simulink library "avl2DLiftingBdy_cl"  (R2018b)
settings: Solver=VariableStepAuto  StartTime=0.0  StopTime=10.0  RelTol=1e-3
values from neighbouring files (symbols this model uses):
  Bref = dsgnData.Bref    [avl2DLiftingBdy_ts.m]
  Cref = dsgnData.Cref    [avl2DLiftingBdy_ts.m]
  grav = 9.81    [avl2DLiftingBdy_ts.m]
  ini_euler = [0;0;0]    [avl2DLiftingBdy_ts.m]
  ini_O_Vcm_o = [0;0;0]    [avl2DLiftingBdy_ts.m]
  ini_OwB = [0;0;0]    [avl2DLiftingBdy_ts.m]
  ini_Rcm_o = [0;0;0]    [avl2DLiftingBdy_ts.m]
  mass = 10    [avl2DLiftingBdy_ts.m]
  MI = eye(3)    [avl2DLiftingBdy_ts.m]
  Rcb_cm = [0;0;0.1]    [avl2DLiftingBdy_ts.m]
  rho_fluid = 1    [avl2DLiftingBdy_ts.m]
  Sref = dsgnData.Sref    [avl2DLiftingBdy_ts.m]
  vol = 20    [avl2DLiftingBdy_ts.m]
undefined symbols (not defined in the file or in its folder): CDtot_2D_Tbl, CLtot_2D_Tbl, Cltot_2D_Tbl, Cmtot_2D_Tbl, Cntot_2D_Tbl, k_CS_gain, m_added, some_class, turbine
libraries: BdyFrameGravForce_ul x1, avlAerodynamics2D x1, bdyFrameBuoyFnM_ul x1, calcAttchPtStates_ul x1, simpleDragTurbine_ul x1, sixDoFDynamics_ul x1, sumAttchPtsFnM_ul x1
settings Model: Creator=Ayaz  LastModifiedBy=asiddiq2

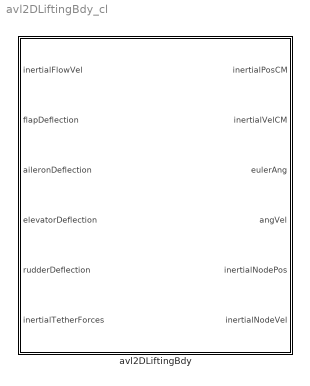
== system avl2DLiftingBdy_cl ==
  avl2DLiftingBdy : Subsystem  mask{M=mass, M_added=m_added, J=MI, vol=vol, Rcb_cm=Rcb_cm, turb_struct=turbine, cls_obj=some_class, g=grav, rho_fluid=rho_fluid, initPos=ini_Rcm_o, initVel=ini_O_Vcm_o, initEulAngs=ini_euler, initAngVel=ini_OwB, CLTable=CLtot_2D_Tbl, CDTable=CDtot_2D_Tbl, CMxTable=Cltot_2D_Tbl, CMyTable=Cmtot_2D_Tbl, CMzTable=Cntot_2D_Tbl, CsGainMatrix=k_CS_gain, CRef=Cref, BRef=Bref, SRef=Sref}
      mask prompts: M "Mass"; M_added "Added Mass Matrix"; J "Inertia matrix"; vol "Body volume"; Rcb_cm "Center of buoyamcy vector"; turb_struct "Turbines structure"; cls_obj "Object consisting variable '.tetherAttchPt'"; g "Gravitational acceleration"; rho_fluid "Fluid density"; initPos "Initial position"; initVel "Initial velocity"; initEulAngs "Initial Euler Angles"; initAngVel "Initial Angular Velocity Vec"; CLTable "CL lookup table object"; CDTable "CD lookup table object"; CMxTable "CMx lookup table object"; CMyTable "CMy lookup table object"; CMzTable "CMz lookup table object"; CsGainMatrix "Control surface gain matrix"; CRef "Pitch Moment Reference Length (AVL Cref)"; BRef "Roll & Yaw Moment Reference Length (AVL Bref)"; SRef "Ref area (AVL Sref)"
      mask TypeOptions M: BdyFrameGravForce/M | sixDoFDynamics1/M
      mask TypeOptions M_added: sixDoFDynamics1/M_added
      mask TypeOptions J: sixDoFDynamics1/J
      mask TypeOptions vol: bdyFrameBuoyForceAndMoment/vol
      mask TypeOptions Rcb_cm: bdyFrameBuoyForceAndMoment/Rcb_cm
      mask TypeOptions turb_struct: simpleDragTurbine/turb_struct
      mask TypeOptions cls_obj: calcAttchPtStates/cls_obj | sumAttchPtsFnM/cls_obj
      mask TypeOptions g: BdyFrameGravForce/g | bdyFrameBuoyForceAndMoment/g
      mask TypeOptions rho_fluid: avlAerodynamics2D/rho_fluid | bdyFrameBuoyForceAndMoment/rho_fluid | simpleDragTurbine/rho_fluid
      mask TypeOptions initPos: sixDoFDynamics1/initPos
      mask TypeOptions initVel: sixDoFDynamics1/initVel
      mask TypeOptions initEulAngs: sixDoFDynamics1/initEulAngs
      mask TypeOptions initAngVel: sixDoFDynamics1/initAngVel
      mask TypeOptions CLTable: avlAerodynamics2D/CLTable
      mask TypeOptions CDTable: avlAerodynamics2D/CDTable
      mask TypeOptions CMxTable: avlAerodynamics2D/CMxTable
      mask TypeOptions CMyTable: avlAerodynamics2D/CMyTable
      mask TypeOptions CMzTable: avlAerodynamics2D/CMzTable
      mask TypeOptions CsGainMatrix: avlAerodynamics2D/CsGainMatrix
      mask TypeOptions CRef: avlAerodynamics2D/CRef
      mask TypeOptions BRef: avlAerodynamics2D/BRef
      mask TypeOptions SRef: avlAerodynamics2D/SRef
      mask DialogControl Container20 Prompt: Parameters
      mask DialogControl ParameterGroupVar Prompt: Physical Parameters
      mask DialogControl Container12 Prompt: Turbine
      mask DialogControl Container13 Prompt: Tether attachment points
      mask DialogControl Container24 Prompt: Environment
      mask DialogControl Container25 Prompt: Initial conditions
      mask DialogControl Container7 Prompt: AVL

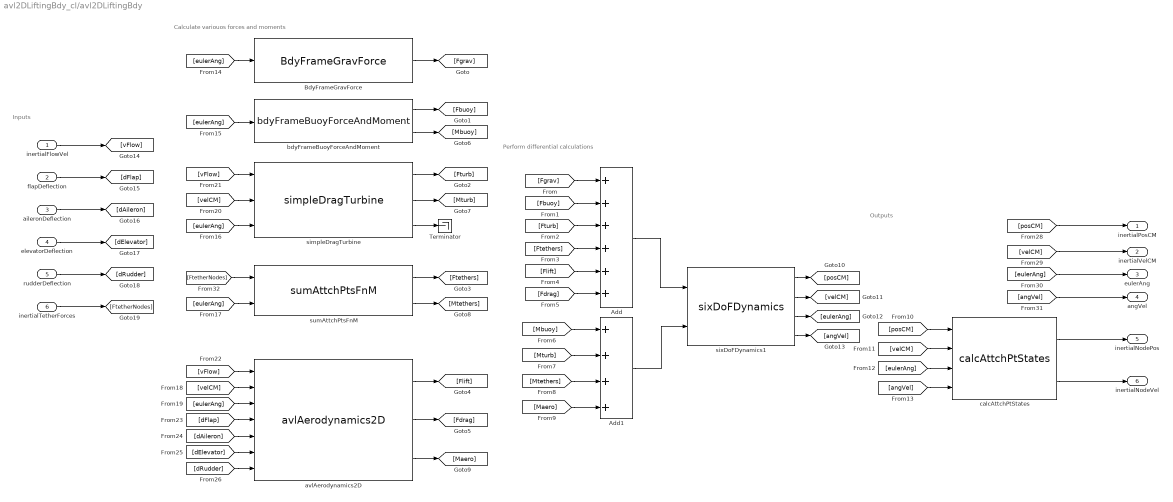
== system avl2DLiftingBdy_cl/avl2DLiftingBdy ==
  note: Outputs
  note: Inputs
  note: Calculate variouos forces and moments
  note: Perform differential calculations
  inertialFlowVel : Inport
  flapDeflection : Inport  Port=2
  aileronDeflection : Inport  Port=3
  elevatorDeflection : Inport  Port=4
  rudderDeflection : Inport  Port=5
  inertialTetherForces : Inport  Port=6
  Add : Sum  Inputs=++++++
  Add1 : Sum  Inputs=++++
  BdyFrameGravForce : BdyFrameGravForce_ul/BdyFrameGravForce  M=M  g=g
  Terminator : Terminator
  avlAerodynamics2D : avlAerodynamics2D/avlAerodynamics2D  CLTable=CLTable  CDTable=CDTable  CMxTable=CMxTable  CMyTable=CMyTable  CMzTable=CMzTable  CsGainMatrix=CsGainMatrix  CRef=CRef  BRef=BRef  SRef=SRef  rho_fluid=rho_fluid
  bdyFrameBuoyForceAndMoment : bdyFrameBuoyFnM_ul/bdyFrameBuoyForceAndMoment  vol=vol  rho_fluid=rho_fluid  g=g  Rcb_cm=Rcb_cm
  calcAttchPtStates : calcAttchPtStates_ul/calcAttchPtStates  cls_obj=cls_obj
  simpleDragTurbine : simpleDragTurbine_ul/simpleDragTurbine  rho_fluid=rho_fluid  turb_struct=turb_struct
  sixDoFDynamics1 : sixDoFDynamics_ul/sixDoFDynamics  M=M  M_added=M_added  J=J  initPos=initPos  initVel=initVel  initEulAngs=initEulAngs  initAngVel=initAngVel
  sumAttchPtsFnM : sumAttchPtsFnM_ul/sumAttchPtsFnM  cls_obj=cls_obj
  inertialPosCM : Outport
  inertialVelCM : Outport  Port=2
  eulerAng : Outport  Port=3
  angVel : Outport  Port=4
  inertialNodePos : Outport  Port=5
  inertialNodeVel : Outport  Port=6
  wires:
  [Mtethers] -> Add1/3
  [velCM] -> avlAerodynamics2D/2
  [angVel] -> calcAttchPtStates/4
  [eulerAng] -> calcAttchPtStates/3
  sixDoFDynamics1/4 -> [angVel]
  sixDoFDynamics1/3 -> [eulerAng]
  [posCM] -> calcAttchPtStates/1
  sixDoFDynamics1/2 -> [velCM]
  [Mturb] -> Add1/2
  [eulerAng] -> sumAttchPtsFnM/2
  [eulerAng] -> bdyFrameBuoyForceAndMoment/1
  [eulerAng] -> BdyFrameGravForce/1
  [Mbuoy] -> Add1/1
  simpleDragTurbine/3 -> Terminator/1
  [Ftethers] -> Add/4
  avlAerodynamics2D/2 -> [Fdrag]
  Add1/1 -> sixDoFDynamics1/2
  avlAerodynamics2D/3 -> [Maero]
  [Fbuoy] -> Add/2
  avlAerodynamics2D/1 -> [Flift]
  sumAttchPtsFnM/1 -> [Ftethers]
  [velCM] -> calcAttchPtStates/2
  [Maero] -> Add1/4
  [Fturb] -> Add/3
  simpleDragTurbine/2 -> [Mturb]
  simpleDragTurbine/1 -> [Fturb]
  [Flift] -> Add/5
  Add/1 -> sixDoFDynamics1/1
  bdyFrameBuoyForceAndMoment/2 -> [Mbuoy]
  [eulerAng] -> avlAerodynamics2D/3
  BdyFrameGravForce/1 -> [Fgrav]
  [Fdrag] -> Add/6
  [Fgrav] -> Add/1
  sumAttchPtsFnM/2 -> [Mtethers]
  bdyFrameBuoyForceAndMoment/1 -> [Fbuoy]
  [eulerAng] -> simpleDragTurbine/3
  [velCM] -> simpleDragTurbine/2
  sixDoFDynamics1/1 -> [posCM]
  inertialFlowVel/1 -> [vFlow]
  [vFlow] -> simpleDragTurbine/1
  [vFlow] -> avlAerodynamics2D/1
  rudderDeflection/1 -> [dRudder]
  elevatorDeflection/1 -> [dElevator]
  aileronDeflection/1 -> [dAileron]
  flapDeflection/1 -> [dFlap]
  [dFlap] -> avlAerodynamics2D/4
  [dAileron] -> avlAerodynamics2D/5
  [dElevator] -> avlAerodynamics2D/6
  [dRudder] -> avlAerodynamics2D/7
  inertialTetherForces/1 -> [FtetherNodes]
  [FtetherNodes] -> sumAttchPtsFnM/1
  [posCM] -> inertialPosCM/1
  [velCM] -> inertialVelCM/1
  [eulerAng] -> eulerAng/1
  [angVel] -> angVel/1
  calcAttchPtStates/2 -> inertialNodeVel/1
  calcAttchPtStates/1 -> inertialNodePos/1
